simulink library "filteredPIDControllerAW_ul"  (R2020a)
settings: Solver=VariableStepAuto  StartTime=0.0  StopTime=10.0  RelTol=1e-3
undefined symbols (not defined in the file): LaRCtrl
settings Model: Creator=mcobb  LastModifiedBy=andre
settings DataIOCC: ReturnWorkspaceOutputs=off
settings DebuggingCC: ArithmeticOperatorsInVariantConditions=warning
settings SFSimCC: CustomCodeUndefinedFunction=UseInterfaceOnly

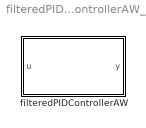
== system filteredPIDControllerAW_ul ==
  filteredPIDControllerAW : Subsystem  mask{kp=LaRCtrl.elevCmd.kp.Value, ki=LaRCtrl.elevCmd.ki.Value, kd=LaRCtrl.elevCmd.kd.Value, tau=LaRCtrl.elevCmd.tau.Value, cmax=LaRCtrl.controlSigMax.upperLimit.Value, cmin=LaRCtrl.controlSigMax.lowerLimit.Value}
      mask prompts: kp "Proportional Gain, kp"; ki "Integral Gain, ki"; kd "Derivative Gain, kd"; tau "Time Constant, s"; cmax "Control Upper Limit"; cmin "Control Lower Limit"

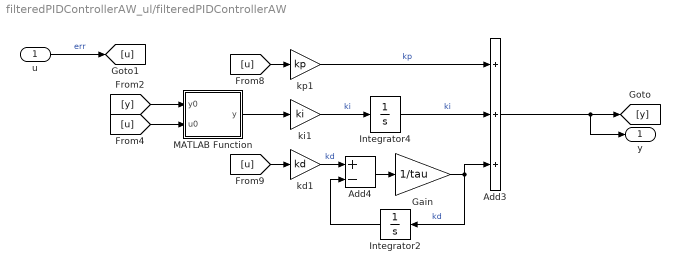
== system filteredPIDControllerAW_ul/filteredPIDControllerAW ==
  u : Inport  PortDimensions=1
  Add3 : Sum  Inputs=+++
  Add4 : Sum  Inputs=+-
  Gain : Gain  Gain=1/tau
  Integrator2 : Integrator  ContinuousStateAttributes='ctrlDerivative'
  Integrator4 : Integrator  ContinuousStateAttributes='ctrlIntegral'
  MATLAB Function : MATLAB Function  TreatAsAtomicUnit=on  mask{cMax=cmax, cMin=cmin}
      mask prompts: cMax "Max control value:"; cMin "Min control value:"
  kd1 : Gain  Gain=kd
  ki1 : Gain  Gain=ki
  kp1 : Gain  Gain=kp
  y : Outport  PortDimensions=1  VectorParamsAs1DForOutWhenUnconnected=off
  wires:
  [u] -> MATLAB Function/2(u0)
  [y] -> MATLAB Function/1(y0)
  u/1 -> [u]  "err"
  kd1/1 -> Add4/1  "kd"
  Integrator2/1 -> Add4/2
  Integrator4/1 -> Add3/2  "ki"
  kp1/1 -> Add3/1  "kp"
  Add4/1 -> Gain/1
  [u] -> kp1/1
  ki1/1 -> Integrator4/1  "ki"
  Gain/1 -> Add3/3, Integrator2/1  "kd"
  [u] -> kd1/1
  MATLAB Function/1(y) -> ki1/1
  Add3/1 -> y/1, [y]

== matlab function filteredPIDControllerAW_ul/filteredPIDControllerAW/MATLAB Function ==
  data: y0 input; u0 input; y output; cMax parameter; cMin parameter
function y = fcn(y0, u0, cMax, cMin)

if y0 > cMax
    y1 = cMax; 
elseif y0 < cMin
    y1 = cMin; 
else
    y1 = y0; 
end

sat = y0-y1; 
aw = exp(-1e5*sat^2); 
y = aw*u0;
